simulink model "radar_missile_system"  (R2025b)
settings: Solver=VariableStepAuto  StartTime=0.0  StopTime=10.0  RelTol=1e-3
libraries: simulink x4

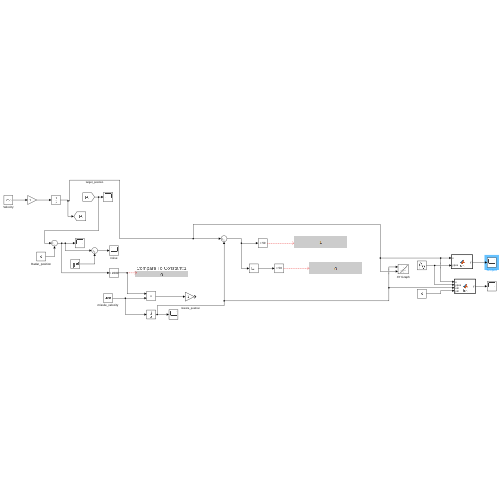
[thumbnail: Simulink's stored preview of the top-level diagram]
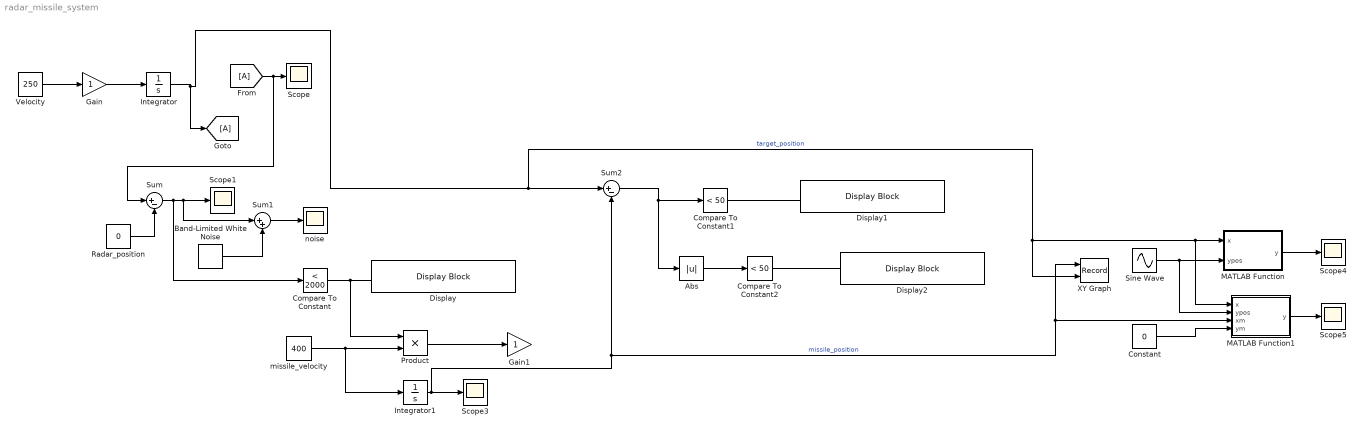
== system radar_missile_system ==
  Abs : Abs  SaturateOnIntegerOverflow=off
  Band-Limited White Noise : simulink/Sources/Band-Limited White Noise  Cov=50  Ts=0.1  seed=[23341]
  Compare To Constant : simulink/Logic and Bit Operations/Compare To Constant  relop=<  const=2000  OutDataTypeStr=boolean
  Compare To Constant1 : simulink/Logic and Bit Operations/Compare To Constant  relop=<  const=50  OutDataTypeStr=boolean
  Compare To Constant2 : simulink/Logic and Bit Operations/Compare To Constant  relop=<  const=50  OutDataTypeStr=boolean
  Constant : Constant  Value=0
  Display : DisplayBlock  Transparency=1  GridColor=[0.502, 0.502, 0.502]
  Display1 : DisplayBlock  LabelPosition=Hide  Transparency=1  GridColor=[0.502, 0.502, 0.502]
  Display2 : DisplayBlock  LabelPosition=Hide  Transparency=1  GridColor=[0.502, 0.502, 0.502]
  From : From
  Gain : Gain
  Gain1 : Gain
  Goto : Goto
  Integrator : Integrator
  Integrator1 : Integrator
  MATLAB Function : MATLAB Function  TreatAsAtomicUnit=on
  MATLAB Function1 : MATLAB Function  TreatAsAtomicUnit=on  SystemSampleTime=0.05
  Product : Product
  Radar_position : Constant  Value=0
  Scope{,1,3..5} (5 alike) : Scope
      Scope settings: ActiveDisplayYMinimum=-557.27188141683769  ActiveDisplayYMaximum=3060.3062435831603
      Scope1 settings: ActiveDisplayYMinimum=-312.50000000000006  ActiveDisplayYMaximum=2812.5000000000009
      Scope3 settings: ActiveDisplayYMinimum=-1399.9225031851374  ActiveDisplayYMaximum=4801.6824180776666  DataLoggingVariableName=ScopeData3
      Scope4 settings: ActiveDisplayYMinimum=-1955.7261628932083  ActiveDisplayYMaximum=4889.4508604525508  DataLoggingVariableName=ScopeData4
      Scope5 settings: ActiveDisplayYMinimum=-49587.767614169818  ActiveDisplayYMaximum=-3190.4323115205625  DataLoggingVariableName=ScopeData5
  Sine Wave : Sin  Amplitude=1000  Bias=1000  Frequency=0.1  SampleTime=0
  Sum : Sum  Inputs=|+-
  Sum1 : Sum  Inputs=|++
  Sum2 : Sum  Inputs=|+-
  Velocity : Constant  Value=250
  XY Graph : Record  NumPorts=2.0  FileSettingsInternal="{\"entries\":[{\"content\":{\"excelSettings\":{\"content\":{},\"type\":\"Streamout.ExcelSettings\"},\"parquetSettings\":{\"content\":{},\"type\":\"Streamout.ParquetSettings\"}},\"type\":\"Streamout.FileSettingStorage\",\"uuid\":\"\"}],\"packageUris\":[\"http:\\/\\/schema.mathworks.com\\/mf0\\/streamout_blocks\\/R2020a\"],\"version\":\"1.0\"}"  FrameSettings=[0, 0]  Layout=[1 1]  SignalsInternal="{\"entries\":[{\"content\":{\"signals\":[{\"content\":{\"blockPath\":[],\"dimensions\":[1],\"domain\":\"\",\"lineColor\":\"#a2142f\",\"plots\":[ 1 ],\"port\":1,\"sid\":[\"\"],\"signalID\":1,\"signalName\":\"missile_position\"},\"type\":\"RecordBlkView.Signal\",\"uuid\":\"\"},{\"content\":{\"blockPath\":[],\"dimensions\":[1],\"domain\":\"\",\"lineColor\":\"#139fff\",\"plots\":[ 1 ],\"port\":2,\"sid\":[\"\"],\"signalID\":2,\"signalName\":\"target_position\"},\"type\":\"RecordBlkView.Signal\",\"uuid\":\"\"}]},\"type\":\"RecordBlkView.InputSignals\",\"uuid\":\"\"}],\"packageUris\":[\"http:\\/\\/schema.mathworks.com\\/mf0\\/streamout_blocks\\/R2020a\"],\"version\":\"1.0\"}"  VisualizationBindings="{\"xyplotplugin\":{\"info\":[{\"series\":[{\"bindingParametersList\":[{\"parameter\":\"X-Axis\",\"signalID\":1,\"signalName\":\"missile_position\"},{\"parameter\":\"Y-Axis\",\"signalID\":2,\"signalName\":\"target_position\"}],\"seriesID\":0}],\"subplotID\":1}]}}"  CompatibilityTag=XY
  missile_velocity : Constant  Value=400
  noise : Scope
      settings: ActiveDisplayYMinimum=-381.84845943592461  ActiveDisplayYMaximum=3294.6557475077525  DataLoggingVariableName=ScopeData2
  wires:
  Velocity/1 -> Gain/1
  Gain/1 -> Integrator/1
  From/1 -> Sum/1, Scope/1
  Radar_position/1 -> Sum/2
  Sum/1 -> Compare To Constant/1, Sum1/1, Scope1/1
  Band-Limited White Noise/1 -> Sum1/2
  Sum1/1 -> noise/1
  Compare To Constant/1 -> Product/1
  Product/1 -> Gain1/1
  missile_velocity/1 -> Integrator1/1, Product/2
  Sum2/1 -> Abs/1, Compare To Constant1/1
  Compare To Constant1/1 -> ?
  Abs/1 -> Compare To Constant2/1
  Compare To Constant2/1 -> ?
  Sine Wave/1 -> MATLAB Function1/2(ypos), MATLAB Function/2(ypos)
  Integrator1/1 -> MATLAB Function1/3(xm), XY Graph/1, Sum2/2, Scope3/1  "missile_position"
  MATLAB Function/1(y) -> Scope4/1
  Integrator/1 -> MATLAB Function1/1(x), MATLAB Function/1(x), XY Graph/2, Sum2/1, Goto/1  "target_position"
  MATLAB Function1/1(y) -> Scope5/1
  Constant/1 -> MATLAB Function1/4(ym)

== matlab function radar_missile_system/MATLAB Function1 ==
  data: x input; y output; ypos input; xm input; ym input
function y = fcn(x,ypos,xm,ym)

persistent fig h_target h_missile sweep_angle sweep_line

if isempty(fig)
    fig = figure(100);
    sweep_angle = 0;
    
    % Radar setup
    theta = linspace(0,2*pi,200);
    
    clf
    hold on
    
    % Range rings
    for r = [1000 2000 3000]
        plot(r*cos(theta), r*sin(theta),'g:')
    end
    
    % Radar boundary
    plot(3000*cos(theta), 3000*sin(theta),'g','LineWidth',1.5)
    
    % Center point
    plot(0,0,'g+')
    
    grid on
    axis equal
    xlim([-3000 3000])
    ylim([-3000 3000])
    
    title('Radar System UI')
    xlabel('X Position')
    ylabel('Y Position')
    
    % Target
    h_target = plot(x,ypos,'ro','MarkerSize',8,'MarkerFaceColor','r');
    
    % Missile
    h_missile = plot(xm,ym,'bo','MarkerSize',8,'MarkerFaceColor','b');
    
    % Sweep line
    sweep_line = plot([0 0],[0 0],'g','LineWidth',1.5);

else
    % Update target
    set(h_target,'XData',x,'YData',ypos);
    
    % Target lock effect
    if sqrt(x^2 + ypos^2) < 2000
        set(h_target,'Color','y','MarkerSize',12) % locked
    else
        set(h_target,'Color','r','MarkerSize',8)
    end
    
    % Update missile
    set(h_missile,'XData',xm,'YData',ym);
end

% --- Radar Sweep ---
sweep_angle = sweep_angle + 0.05;

r = 3000;

% Sweep trail
for i = 1:5
    angle = sweep_angle - i*0.1;
    plot([0 r*cos(angle)], [0 r*sin(angle)], 'g')
end

% Main sweep
x_sweep = [0 r*cos(sweep_angle)];
y_sweep = [0 r*sin(sweep_angle)];

set(sweep_line,'XData',x_sweep,'YData',y_sweep);

% --- Interception Detection ---
if abs(x - xm) < 50 && abs(ypos - ym) < 50
    plot(x,ypos,'rx','MarkerSize',20,'LineWidth',3)
    text(x,ypos,'HIT','Color','red','FontSize',12)
end

% --- Live Data ---
text(-2800,2800,['Target X: ', num2str(x)])
text(-2800,2500,['Target Y: ', num2str(ypos)])

drawnow limitrate

y = x;

== matlab function radar_missile_system/MATLAB Function ==
  data: x input; y output; ypos input
function y = fcn(x,ypos)

persistent fig

if isempty(fig)
    fig = figure;
end

figure(fig)
plot(x,ypos,'ro','MarkerSize',8,'MarkerFaceColor','r')
grid on
xlim([0 6000])
ylim([0 2000])

xlabel('X Position')
ylabel('Y Position')
title('Radar Target Tracking')

drawnow

y = x;
